simulink model "pure_pursuit_sl"  (R2019a)
settings: Solver=FixedStepDiscrete  StartTime=0.0  StopTime=inf  FixedStep=0.01  RelTol=1e-3
model workspace (MAT data in the model file):
  SL_ROS_VariableLengthArrays_MaxSizes : struct (value not decoded)
  MCOS : class17 (value not decoded)
  MCOS : class17 (value not decoded)
  MCOS : class17 (value not decoded)
  MCOS : class17 (value not decoded)
undefined symbols (not defined in the file): Action, Color, Colors, Colors_SL_Info, FrameLocked, Header, Id, Ns, Points, Points_SL_Info, Pose, Scale, Twist, Type, X, Y, Z
libraries: robotlib x22, robotcorelib x4, simulink x1
(part 2 of 2)

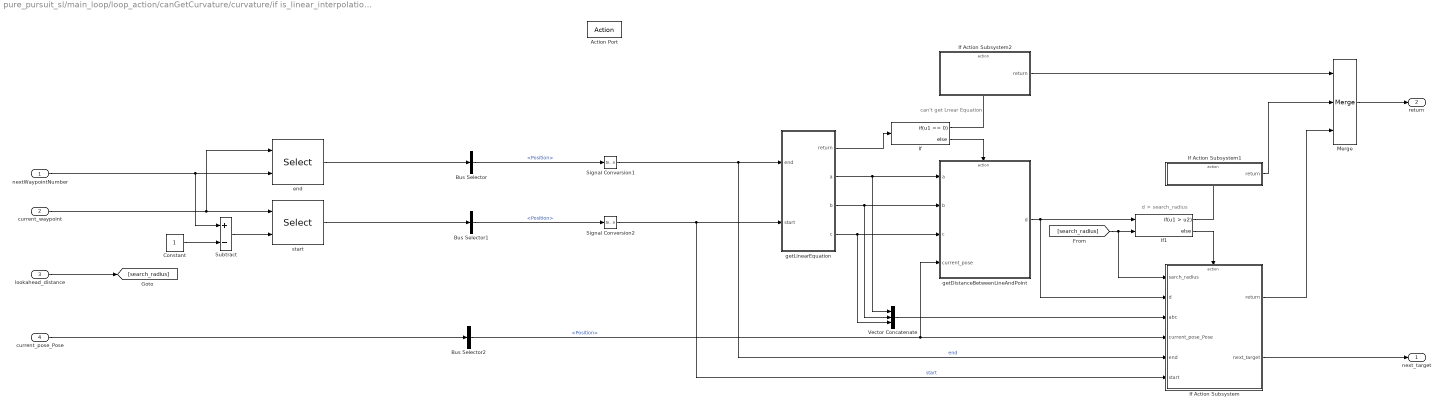
== system pure_pursuit_sl/main_loop/loop_action/canGetCurvature/curvature/if is_linear_interpolation_ is false or next waypoint is first or last/interpolateNextTarget/Subsystem ==
  note: d > search_radius
  note: can't get Lnear Equation
  nextWaypointNumber : Inport
  current_waypoint : Inport  Port=2
  lookahead_distance : Inport  Port=3
  current_pose_Pose : Inport  Port=4
  Action Port : ActionPort  ActionPortLabel=else
  Bus Selector : BusSelector  OutputSignals=Pose.Pose.Position
  Bus Selector1 : BusSelector  OutputSignals=Pose.Pose.Position
  Bus Selector2 : BusSelector  OutputSignals=Position
  Constant : Constant
  If : If  IfExpression=u1 == 0
  If Action Subsystem : Subsystem  TreatAsAtomicUnit=on
  If Action Subsystem1 : Subsystem  TreatAsAtomicUnit=on
  If Action Subsystem2 : Subsystem  TreatAsAtomicUnit=on
  If1 : If  NumInputs=2  IfExpression=u1 > u2
  Merge : Merge  Inputs=3
  Signal Conversion1 : SignalConversion  OverrideOpt=off
  Signal Conversion2 : SignalConversion  OverrideOpt=off
  Subtract : Sum  Inputs=+-
  Vector Concatenate : Concatenate  NumInputs=3
  end : Selector  InputPortWidth=101  IndexOptions=Index vector (port)  Indices=[1 3]  OutputSizes=1
  getDistanceBetweenLineAndPoint : Subsystem  TreatAsAtomicUnit=on
  getLinearEquation : Subsystem  TreatAsAtomicUnit=on
  start : Selector  InputPortWidth=101  IndexOptions=Index vector (port)  Indices=[1 3]  OutputSizes=1
  next_target : Outport
  return : Outport  Port=2
  wires:
  [search_radius] -> If Action Subsystem/1(sarch_radius), If1/2
  Bus Selector/1 -> Signal Conversion1/1  "<Position>"
  start/1 -> Bus Selector1/1
  If Action Subsystem/2(next_target) -> next_target/1
  Signal Conversion2/1 -> getLinearEquation/2(start), If Action Subsystem/6(start)  "start"
  getLinearEquation/3(b) -> Vector Concatenate/2, getDistanceBetweenLineAndPoint/2(b)
  If/2 -> getDistanceBetweenLineAndPoint/Action
  nextWaypointNumber/1 -> Subtract/1, end/2
  current_waypoint/1 -> end/1, start/1
  getDistanceBetweenLineAndPoint/1(d) -> If1/1, If Action Subsystem/2(d)
  Bus Selector2/1 -> getDistanceBetweenLineAndPoint/4(current_pose), If Action Subsystem/4(current_pose_Pose)  "<Position>"
  Merge/1 -> return/1
  If1/1 -> If Action Subsystem1/Action
  getLinearEquation/1(return) -> If/1
  getLinearEquation/4(c) -> Vector Concatenate/3, getDistanceBetweenLineAndPoint/3(c)
  Vector Concatenate/1 -> If Action Subsystem/3(abc)
  getLinearEquation/2(a) -> Vector Concatenate/1, getDistanceBetweenLineAndPoint/1(a)
  Signal Conversion1/1 -> getLinearEquation/1(end), If Action Subsystem/5(end)  "end"
  If1/2 -> If Action Subsystem/Action
  Subtract/1 -> start/2
  If Action Subsystem1/1(return) -> Merge/2
  Bus Selector1/1 -> Signal Conversion2/1  "<Position>"
  lookahead_distance/1 -> [search_radius]
  Constant/1 -> Subtract/2
  If/1 -> If Action Subsystem2/Action
  end/1 -> Bus Selector/1
  If Action Subsystem2/1(return) -> Merge/1
  If Action Subsystem/1(return) -> Merge/3
  current_pose_Pose/1 -> Bus Selector2/1

== system pure_pursuit_sl/main_loop/loop_action/canGetCurvature/curvature/if is_linear_interpolation_ is false or next waypoint is first or last/ next_waypoint_is_first_or_last/calcCurvature/calcRelativeCoordinate ==
  target : Inport
  current_pose_ : Inport  Port=2
  Bus Selector : BusSelector  OutputSignals=Orientation.W,Orientation.X,Orientation.Y,Orientation.Z
  Bus Selector1 : BusSelector  OutputSignals=Position.X,Position.Y,Position.Z
  Bus Selector3 : BusSelector  OutputSignals=X,Y,Z
  Constant : Constant
  Coordinate Transformation Conversion : robotcorelib/Coordinate Transformation Conversion  InputRepresentation=Quaternion  InputEulerSequence=XYZ  ShowTrVecInputPort=on  OutputRepresentation=Homogeneous Transformation  OutputEulerSequence=ZYX  ShowTrVecOutputPort=on  SimulateUsing=Interpreted execution
      settings: SourceProductBaseCode=RO
  Position Vector : Concatenate  NumInputs=3
  Product : Product  Inputs=/  Multiplication=Matrix(*)
  Product1 : Product  Multiplication=Matrix(*)
  "Quaternion Vector " : Concatenate  NumInputs=4
  point : Concatenate  NumInputs=4
  ros_pose : Outport
  wires:
  current_pose_/1 -> Bus Selector/1, Bus Selector1/1
  Position Vector/1 -> Coordinate Transformation Conversion/2
  Bus Selector1/3 -> Position Vector/3  "<Z>"
  "Quaternion Vector "/1 -> Coordinate Transformation Conversion/1
  Bus Selector1/2 -> Position Vector/2  "<Y>"
  Bus Selector1/1 -> Position Vector/1  "<X>"
  Coordinate Transformation Conversion/1 -> Product/1
  Product/1 -> Product1/1
  target/1 -> Bus Selector3/1
  Bus Selector3/2 -> point/2  "<Y>"
  Bus Selector3/3 -> point/3  "<Z>"
  Bus Selector3/1 -> point/1  "<X>"
  point/1 -> Product1/2
  Product1/1 -> ros_pose/1  "ros_pose"
  Bus Selector/1 -> "Quaternion Vector "/1  "<W>"
  Bus Selector/2 -> "Quaternion Vector "/2  "<X>"
  Bus Selector/3 -> "Quaternion Vector "/3  "<Y>"
  Bus Selector/4 -> "Quaternion Vector "/4  "<Z>"
  Constant/1 -> point/4

== system pure_pursuit_sl/main_loop/loop_action/canGetCurvature/curvature/if is_linear_interpolation_ is false or next waypoint is first or last/ next_waypoint_is_first_or_last/calcCurvature/getPlaneDistance ==
  target1 : Inport
  target2 : Inport  Port=2
  Add : Sum
  Bus Selector1 : BusSelector  OutputSignals=Position.X,Position.Y
  Bus Selector2 : BusSelector  OutputSignals=X,Y
  Math Function : Math  Operator=square  SaturateOnIntegerOverflow=on
  Math Function1 : Math  Operator=square  SaturateOnIntegerOverflow=on
  Sqrt : Sqrt  SaturateOnIntegerOverflow=on
  Subtract : Sum  Inputs=+-
  Subtract1 : Sum  Inputs=+-
  Distance : Outport
  wires:
  Subtract1/1 -> Math Function/1
  target2/1 -> Bus Selector1/1
  Bus Selector1/1 -> Subtract1/2  "<X>"
  target1/1 -> Bus Selector2/1
  Add/1 -> Sqrt/1
  Bus Selector2/1 -> Subtract1/1  "<X>"
  Bus Selector2/2 -> Subtract/1  "<Y>"
  Sqrt/1 -> Distance/1
  Math Function/1 -> Add/1
  Subtract/1 -> Math Function1/1
  Math Function1/1 -> Add/2
  Bus Selector1/2 -> Subtract/2  "<Y>"

== system pure_pursuit_sl/main_loop/loop_action/canGetCurvature/curvature/if is_linear_interpolation_ is false or next waypoint is first or last/ next_waypoint_is_first_or_last/calcCurvature/minus_KAPPA_MIN ==
  In1 : Inport
  Action Port : ActionPort  ActionPortLabel=else
  Unary Minus : UnaryMinus
  Out1 : Outport
  wires:
  In1/1 -> Unary Minus/1
  Unary Minus/1 -> Out1/1

== system pure_pursuit_sl/main_loop/loop_action/canGetCurvature/curvature/if is_linear_interpolation_ is false or next waypoint is first or last/ next_waypoint_is_first_or_last/calcCurvature/num_div_den ==
  denominator : Inport
  numerator : Inport  Port=2
  Action Port : ActionPort  ActionPortLabel=if(u1 ~= 0)
  Divide : Product  Inputs=*/
  kappa : Outport
  wires:
  denominator/1 -> Divide/2
  numerator/1 -> Divide/1
  Divide/1 -> kappa/1

== system pure_pursuit_sl/main_loop/loop_action/canGetCurvature/curvature/if is_linear_interpolation_ is false or next waypoint is first or last/ next_waypoint_is_first_or_last/calcCurvature/plus_KAPPA_MIN ==
  In1 : Inport
  Action Port : ActionPort  ActionPortLabel=elseif(u2 > 0)
  Out1 : Outport
  wires:
  In1/1 -> Out1/1

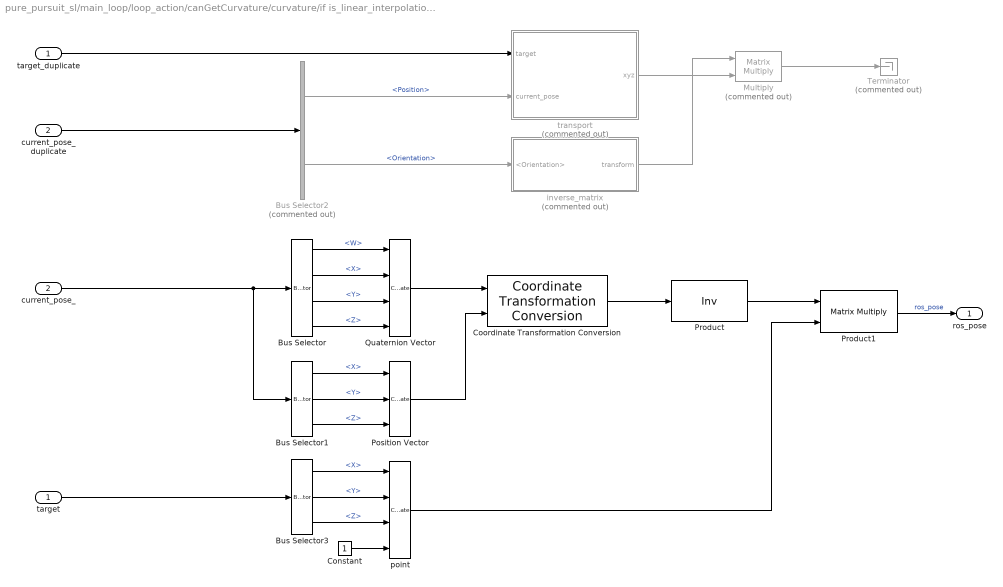
== system pure_pursuit_sl/main_loop/loop_action/canGetCurvature/curvature/if is_linear_interpolation_ is false or next waypoint is first or last/calcCurvature/calcCurvature/calcRelativeCoordinate ==
  target : Inport
  current_pose_ : Inport  Port=2
  Bus Selector : BusSelector  OutputSignals=Orientation.W,Orientation.X,Orientation.Y,Orientation.Z
  Bus Selector1 : BusSelector  OutputSignals=Position.X,Position.Y,Position.Z
  Bus Selector2 : BusSelector  Commented=on  OutputSignals=Position,Orientation
  Bus Selector3 : BusSelector  OutputSignals=X,Y,Z
  Constant : Constant
  Coordinate Transformation Conversion : robotcorelib/Coordinate Transformation Conversion  InputRepresentation=Quaternion  InputEulerSequence=XYZ  ShowTrVecInputPort=on  OutputRepresentation=Homogeneous Transformation  OutputEulerSequence=ZYX  ShowTrVecOutputPort=on  SimulateUsing=Interpreted execution
      settings: SourceProductBaseCode=RO
  Multiply : Product  Commented=on  Multiplication=Matrix(*)
  Position Vector : Concatenate  NumInputs=3
  Product : Product  Inputs=/  Multiplication=Matrix(*)
  Product1 : Product  Multiplication=Matrix(*)
  "Quaternion Vector " : Concatenate  NumInputs=4
  Terminator : Terminator  Commented=on
  current_pose_duplicate : InportShadow  Port=2
  inverse_matrix : Subsystem  Commented=on
  point : Concatenate  NumInputs=4
  target_duplicate : InportShadow
  transport : Subsystem  Commented=on
  ros_pose : Outport
  wires:
  Bus Selector2/2 -> inverse_matrix/1(<Orientation>)  "<Orientation>"
  transport/1(xyz) -> Multiply/2
  inverse_matrix/1(transform) -> Multiply/1
  target_duplicate/1 -> transport/1(target)
  Multiply/1 -> Terminator/1
  current_pose_/1 -> Bus Selector/1, Bus Selector1/1
  Bus Selector2/1 -> transport/2(current_pose)  "<Position>"
  Position Vector/1 -> Coordinate Transformation Conversion/2
  Bus Selector1/3 -> Position Vector/3  "<Z>"
  "Quaternion Vector "/1 -> Coordinate Transformation Conversion/1
  Bus Selector1/2 -> Position Vector/2  "<Y>"
  Bus Selector1/1 -> Position Vector/1  "<X>"
  Coordinate Transformation Conversion/1 -> Product/1
  current_pose_duplicate/1 -> Bus Selector2/1
  Product/1 -> Product1/1
  target/1 -> Bus Selector3/1
  Bus Selector3/2 -> point/2  "<Y>"
  Bus Selector3/3 -> point/3  "<Z>"
  Bus Selector3/1 -> point/1  "<X>"
  point/1 -> Product1/2
  Product1/1 -> ros_pose/1  "ros_pose"
  Bus Selector/1 -> "Quaternion Vector "/1  "<W>"
  Bus Selector/2 -> "Quaternion Vector "/2  "<X>"
  Bus Selector/3 -> "Quaternion Vector "/3  "<Y>"
  Bus Selector/4 -> "Quaternion Vector "/4  "<Z>"
  Constant/1 -> point/4

== system pure_pursuit_sl/main_loop/loop_action/canGetCurvature/curvature/if is_linear_interpolation_ is false or next waypoint is first or last/calcCurvature/calcCurvature/getPlaneDistance ==
  target1 : Inport
  target2 : Inport  Port=2
  Add : Sum
  Bus Selector1 : BusSelector  OutputSignals=Position.X,Position.Y
  Bus Selector2 : BusSelector  OutputSignals=X,Y
  Math Function : Math  Operator=square  SaturateOnIntegerOverflow=on
  Math Function1 : Math  Operator=square  SaturateOnIntegerOverflow=on
  Sqrt : Sqrt  SaturateOnIntegerOverflow=on
  Subtract : Sum  Inputs=+-
  Subtract1 : Sum  Inputs=+-
  Distance : Outport
  wires:
  Subtract1/1 -> Math Function/1
  target2/1 -> Bus Selector1/1
  Bus Selector1/1 -> Subtract1/2  "<X>"
  target1/1 -> Bus Selector2/1
  Add/1 -> Sqrt/1
  Bus Selector2/1 -> Subtract1/1  "<X>"
  Bus Selector2/2 -> Subtract/1  "<Y>"
  Sqrt/1 -> Distance/1
  Math Function/1 -> Add/1
  Subtract/1 -> Math Function1/1
  Math Function1/1 -> Add/2
  Bus Selector1/2 -> Subtract/2  "<Y>"

== system pure_pursuit_sl/main_loop/loop_action/canGetCurvature/curvature/if is_linear_interpolation_ is false or next waypoint is first or last/calcCurvature/calcCurvature/minus_KAPPA_MIN ==
  In1 : Inport
  Action Port : ActionPort  ActionPortLabel=else
  Unary Minus : UnaryMinus
  Out1 : Outport
  wires:
  In1/1 -> Unary Minus/1
  Unary Minus/1 -> Out1/1

== system pure_pursuit_sl/main_loop/loop_action/canGetCurvature/curvature/if is_linear_interpolation_ is false or next waypoint is first or last/calcCurvature/calcCurvature/num_div_den ==
  denominator : Inport
  numerator : Inport  Port=2
  Action Port : ActionPort  ActionPortLabel=if(u1 ~= 0)
  Divide : Product  Inputs=*/
  kappa : Outport
  wires:
  denominator/1 -> Divide/2
  numerator/1 -> Divide/1
  Divide/1 -> kappa/1

== system pure_pursuit_sl/main_loop/loop_action/canGetCurvature/curvature/if is_linear_interpolation_ is false or next waypoint is first or last/calcCurvature/calcCurvature/plus_KAPPA_MIN ==
  In1 : Inport
  Action Port : ActionPort  ActionPortLabel=elseif(u2 > 0)
  Out1 : Outport
  wires:
  In1/1 -> Out1/1

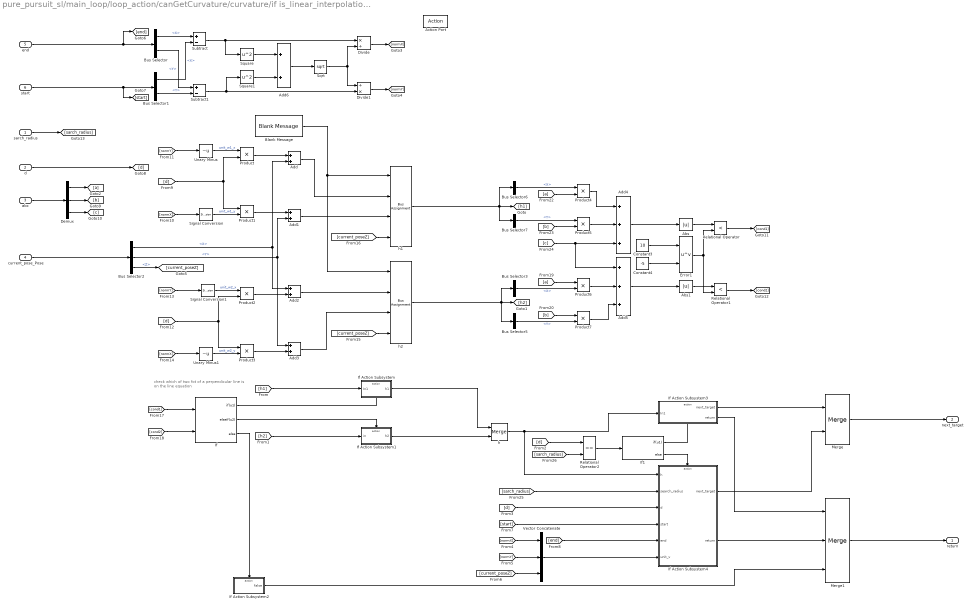
== system pure_pursuit_sl/main_loop/loop_action/canGetCurvature/curvature/if is_linear_interpolation_ is false or next waypoint is first or last/interpolateNextTarget/Subsystem/If Action Subsystem ==
  note: check which of two fot of a perpendicular line
      | is on the line equation
  sarch_radius : Inport
  d : Inport  Port=2
  abc : Inport  Port=3
  current_pose_Pose : Inport  Port=4
  end : Inport  Port=5
  start : Inport  Port=6
  Action Port : ActionPort  ActionPortLabel=else
  Abs : Abs
  Abs1 : Abs
  Add{,1..3,6} (5 alike) : Sum
  Add4 : Sum  Inputs=+++
  Add5 : Sum  Inputs=+++
  Blank Message : robotlib/Blank Message  messageClass=Message  entityType=geometry_msgs/Point  messageType=geometry_msgs/Point  SampleTime=inf
      settings: SourceProductBaseCode=RO
  Bus Selector : BusSelector  OutputSignals=X,Y
  Bus Selector1 : BusSelector  OutputSignals=X,Y
  Bus Selector2 : BusSelector  OutputSignals=X,Y,Z
  Bus Selector3 : BusSelector  OutputSignals=X
  Bus Selector5 : BusSelector  OutputSignals=Y
  Bus Selector6 : BusSelector  OutputSignals=X
  Bus Selector7 : BusSelector  OutputSignals=Y
  Constant3 : Constant  Value=10  OutDataTypeStr=double
  Constant4 : Constant  Value=-5  OutDataTypeStr=double
  Demux : Demux  Outputs=3
  Divide : Product  Inputs=*/
  Divide1 : Product  Inputs=/*
  Error1 : Math  Operator=pow  SaturateOnIntegerOverflow=on
  If : If  NumInputs=2  IfExpression=u1  ElseIfExpressions=u2
  If Action Subsystem : Subsystem  TreatAsAtomicUnit=on
  If Action Subsystem1 : Subsystem  TreatAsAtomicUnit=on
  If Action Subsystem2 : Subsystem  TreatAsAtomicUnit=on
  If Action Subsystem3 : Subsystem  TreatAsAtomicUnit=on
  If Action Subsystem4 : Subsystem  Description=|  TreatAsAtomicUnit=on
      | if there are two intersection
      | get intersection in front of vehicle
      settings: AttributesFormatString=%<Description>
  If1 : If  IfExpression=u1
  Merge : Merge
  Merge1 : Merge  Inputs=3
  Product{,1..7} (8 alike) : Product
  Relational Operator : RelationalOperator  Operator=<  OutDataTypeStr=boolean  RndMeth=Simplest
  Relational Operator1 : RelationalOperator  Operator=<  OutDataTypeStr=boolean  RndMeth=Simplest
  Relational Operator2 : RelationalOperator  Operator===  OutDataTypeStr=boolean  RndMeth=Simplest
  Signal Conversion : SignalConversion  OverrideOpt=off
  Signal Conversion1 : SignalConversion  OverrideOpt=off
  Sqrt : Sqrt  SaturateOnIntegerOverflow=on
  Square : Math  Operator=square  SaturateOnIntegerOverflow=on
  Square1 : Math  Operator=square  SaturateOnIntegerOverflow=on
  Subtract : Sum  Inputs=+-
  Subtract1 : Sum  Inputs=+-
  Unary Minus : UnaryMinus
  Unary Minus1 : UnaryMinus
  Vector Concatenate : Concatenate  NumInputs=3
  h : Merge
  h1 : BusAssignment  AssignedSignals=X,Y,Z
  h2 : BusAssignment  AssignedSignals=X,Y,Z
  return : Outport
  next_target : Outport  Port=2
  wires:
  Bus Selector/2 -> Subtract1/1  "<Y>"
  end/1 -> [end], Bus Selector/1
  start/1 -> [start], Bus Selector1/1
  Bus Selector/1 -> Subtract/1  "<X>"
  Bus Selector1/1 -> Subtract/2  "<X>"
  Bus Selector1/2 -> Subtract1/2  "<Y>"
  [normX] -> Signal Conversion/1
  [normY] -> Unary Minus/1
  Unary Minus/1 -> Product/1  "unit_w1_x"
  current_pose_Pose/1 -> Bus Selector2/1
  Bus Selector2/1 -> Add2/1, Add/2  "<X>"
  Blank Message/1 -> h1/1, h2/1
  Bus Selector2/3 -> [current_poseZ]  "<Z>"
  Product/1 -> Add/1
  [d] -> Product1/1, Product/2
  Product1/1 -> Add1/1
  Bus Selector2/2 -> Add3/1, Add1/2  "<Y>"
  Product2/1 -> Add2/2
  Product3/1 -> Add3/2
  Add/1 -> h1/2
  Add1/1 -> h1/3
  Add2/1 -> h2/2
  Add3/1 -> h2/3
  Bus Selector6/1 -> Product4/1  "<X>"
  [a] -> Product6/1
  Bus Selector7/1 -> Product5/1  "<Y>"
  [b] -> Product7/1
  Product4/1 -> Add4/1
  Product5/1 -> Add4/2
  [c] -> Add5/1, Add4/3
  Bus Selector3/1 -> Product6/2  "<X>"
  Bus Selector5/1 -> Product7/2  "<Y>"
  Product6/1 -> Add5/2
  Product7/1 -> Add5/3
  Constant4/1 -> Error1/2
  Constant3/1 -> Error1/1
  Add4/1 -> Abs/1
  Add5/1 -> Abs1/1
  If/1 -> If Action Subsystem/Action
  If/2 -> If Action Subsystem1/Action
  [h1] -> If Action Subsystem/1(In1)
  [h2] -> If Action Subsystem1/1(in)
  If/3 -> If Action Subsystem2/Action
  If Action Subsystem/1(h1) -> h/1
  If Action Subsystem1/1("h2 ") -> h/2
  sarch_radius/1 -> [sarch_radius]
  [d] -> Relational Operator2/1
  If1/1 -> If Action Subsystem3/Action
  h/1 -> If Action Subsystem3/1(In1), If Action Subsystem4/1(h)
  If1/2 -> If Action Subsystem4/Action
  [d] -> If Action Subsystem4/3(d)
  [normY] -> Vector Concatenate/2
  [normX] -> Vector Concatenate/1
  [current_poseZ] -> Vector Concatenate/3
  Vector Concatenate/1 -> If Action Subsystem4/6(unit_v)
  [start] -> If Action Subsystem4/4(start)
  [end] -> If Action Subsystem4/5("end ")
  If Action Subsystem3/1(next_target) -> Merge/1
  If Action Subsystem4/1(next_target) -> Merge/2
  If Action Subsystem4/2(return) -> Merge1/2
  If Action Subsystem3/2(return) -> Merge1/1
  If Action Subsystem2/1(false) -> Merge1/3
  Merge/1 -> next_target/1
  Merge1/1 -> return/1
  d/1 -> [d]
  Subtract1/1 -> Square1/1, Divide1/2
  Square/1 -> Add6/1
  Subtract/1 -> Square/1, Divide/1
  Square1/1 -> Add6/2
  Add6/1 -> Sqrt/1
  Sqrt/1 -> Divide/2, Divide1/1
  Divide/1 -> [normX]
  Divide1/1 -> [normY]
  Signal Conversion/1 -> Product1/2  "unit_w1_y"
  [d] -> Product3/1, Product2/2
  Unary Minus1/1 -> Product3/2  "unit_w2_y"
  Signal Conversion1/1 -> Product2/1  "unit_w2_x"
  [normY] -> Signal Conversion1/1
  [normX] -> Unary Minus1/1
  [current_poseZ] -> h2/4
  [current_poseZ] -> h1/4
  h1/1 -> Bus Selector6/1, Bus Selector7/1, [h1]
  abc/1 -> Demux/1
  Demux/1 -> [a]
  Demux/2 -> [b]
  Demux/3 -> [c]
  [a] -> Product4/2
  [b] -> Product5/2
  h2/1 -> Bus Selector5/1, [h2], Bus Selector3/1
  Abs/1 -> Relational Operator/1
  Error1/1 -> Relational Operator1/2, Relational Operator/2
  Abs1/1 -> Relational Operator1/1
  Relational Operator/1 -> [cond1]
  Relational Operator1/1 -> [cond2]
  [cond1] -> If/1
  [cond2] -> If/2
  [sarch_radius] -> If Action Subsystem4/2(search_radius)
  [sarch_radius] -> Relational Operator2/2
  Relational Operator2/1 -> If1/1

== system pure_pursuit_sl/main_loop/loop_action/canGetCurvature/curvature/if is_linear_interpolation_ is false or next waypoint is first or last/interpolateNextTarget/Subsystem/If Action Subsystem1 ==
  Action Port : ActionPort  ActionPortLabel=if(u1 > u2)
  Constant1 : Constant  Value=false  OutDataTypeStr=boolean
  return : Outport  InitialOutput=false
  wires:
  Constant1/1 -> return/1

== system pure_pursuit_sl/main_loop/loop_action/canGetCurvature/curvature/if is_linear_interpolation_ is false or next waypoint is first or last/interpolateNextTarget/Subsystem/If Action Subsystem2 ==
  Action Port : ActionPort  ActionPortLabel=if(u1 == 0)
  Constant1 : Constant  Value=false  OutDataTypeStr=boolean
  return : Outport  InitialOutput=false
  wires:
  Constant1/1 -> return/1

== system pure_pursuit_sl/main_loop/loop_action/canGetCurvature/curvature/if is_linear_interpolation_ is false or next waypoint is first or last/interpolateNextTarget/Subsystem/getDistanceBetweenLineAndPoint ==
  a : Inport
  b : Inport  Port=2
  c : Inport  Port=3
  current_pose : Inport  Port=4
  Action Port : ActionPort  ActionPortLabel=else
  Abs : Abs
  Add : Sum  Inputs=+++
  Add1 : Sum
  Bus Selector1 : BusSelector  OutputSignals=X,Y
  Divide : Product  Inputs=*/
  Product : Product
  Product1 : Product
  Sqrt : Sqrt  SaturateOnIntegerOverflow=on
  Square : Math  Operator=square  SaturateOnIntegerOverflow=on
  Square1 : Math  Operator=square  SaturateOnIntegerOverflow=on
  d : Outport
  wires:
  a/1 -> Product/2, Square/1
  current_pose/1 -> Bus Selector1/1
  Bus Selector1/1 -> Product/1  "<X>"
  b/1 -> Product1/2, Square1/1
  Bus Selector1/2 -> Product1/1  "<Y>"
  Product/1 -> Add/2
  Product1/1 -> Add/3
  Add1/1 -> Sqrt/1
  Square/1 -> Add1/1
  Square1/1 -> Add1/2
  Add/1 -> Abs/1
  Sqrt/1 -> Divide/2
  Divide/1 -> d/1
  Abs/1 -> Divide/1
  c/1 -> Add/1

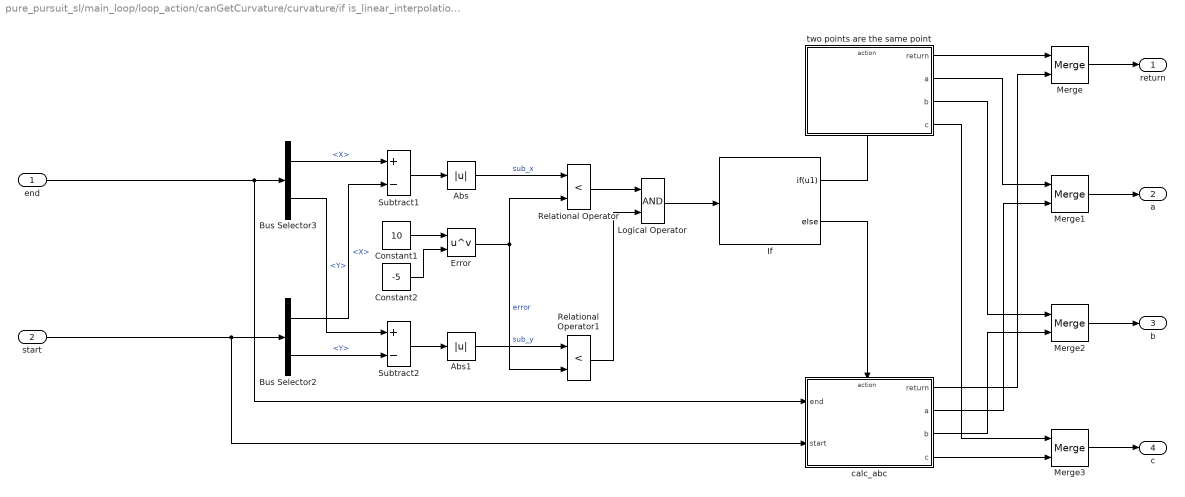
== system pure_pursuit_sl/main_loop/loop_action/canGetCurvature/curvature/if is_linear_interpolation_ is false or next waypoint is first or last/interpolateNextTarget/Subsystem/getLinearEquation ==
  end : Inport
  start : Inport  Port=2
  Abs : Abs
  Abs1 : Abs
  Bus Selector2 : BusSelector  OutputSignals=X,Y
  Bus Selector3 : BusSelector  OutputSignals=X,Y
  Constant1 : Constant  Value=10  OutDataTypeStr=double
  Constant2 : Constant  Value=-5  OutDataTypeStr=double
  Error : Math  Operator=pow  SaturateOnIntegerOverflow=on
  If : If  IfExpression=u1
  Logical Operator : Logic  AllPortsSameDT=off  OutDataTypeStr=boolean
  Merge{,1..3} (4 alike) : Merge
  Relational Operator : RelationalOperator  Operator=<  OutDataTypeStr=boolean  RndMeth=Simplest
  Relational Operator1 : RelationalOperator  Operator=<  OutDataTypeStr=boolean  RndMeth=Simplest
  Subtract1 : Sum  Inputs=+-
  Subtract2 : Sum  Inputs=+-
  calc_abc : Subsystem  TreatAsAtomicUnit=on
  two points are the same point : Subsystem  TreatAsAtomicUnit=on
  return : Outport
  a : Outport  Port=2
  b : Outport  Port=3
  c : Outport  Port=4
  wires:
  Error/1 -> Relational Operator1/2, Relational Operator/2  "error"
  two points are the same point/1(return) -> Merge/1
  Bus Selector3/2 -> Subtract2/1  "<Y>"
  If/2 -> calc_abc/Action
  Merge/1 -> return/1
  Abs1/1 -> Relational Operator1/1  "sub_y"
  Bus Selector2/1 -> Subtract1/2  "<X>"
  Abs/1 -> Relational Operator/1  "sub_x"
  Subtract1/1 -> Abs/1
  calc_abc/1(return) -> Merge/2
  If/1 -> two points are the same point/Action
  start/1 -> Bus Selector2/1, calc_abc/2(start)
  Bus Selector3/1 -> Subtract1/1  "<X>"
  Subtract2/1 -> Abs1/1
  Bus Selector2/2 -> Subtract2/2  "<Y>"
  end/1 -> Bus Selector3/1, calc_abc/1(end)
  Constant2/1 -> Error/2
  Constant1/1 -> Error/1
  Relational Operator/1 -> Logical Operator/1
  Relational Operator1/1 -> Logical Operator/2
  Logical Operator/1 -> If/1
  Merge3/1 -> c/1
  calc_abc/4(c) -> Merge3/2
  two points are the same point/4(c) -> Merge3/1
  two points are the same point/2(a) -> Merge1/1
  calc_abc/2(a) -> Merge1/2
  Merge1/1 -> a/1
  Merge2/1 -> b/1
  two points are the same point/3(b) -> Merge2/1
  calc_abc/3(b) -> Merge2/2

== system pure_pursuit_sl/main_loop/loop_action/canGetCurvature/curvature/if is_linear_interpolation_ is false or next waypoint is first or last/calcCurvature/calcCurvature/calcRelativeCoordinate/inverse_matrix ==
  <Orientation> : Inport
  Bus Creator : BusCreator  Inputs=4
  Bus Selector1 : BusSelector  OutputSignals=W,X,Y,Z
  Bus to Vector : BusToVector
  Coordinate Transformation Conversion : robotcorelib/Coordinate Transformation Conversion  InputRepresentation=Quaternion  InputEulerSequence=ZYX  ShowTrVecInputPort=on  OutputRepresentation=Rotation Matrix  OutputEulerSequence=ZYX  ShowTrVecOutputPort=on  SimulateUsing=Interpreted execution
      settings: SourceProductBaseCode=RO
  inverse : MATLAB Function  TreatAsAtomicUnit=on
  transform : Outport
  wires:
  Coordinate Transformation Conversion/1 -> inverse/1(u)
  inverse/1(y) -> transform/1
  Bus Selector1/3 -> Bus Creator/3  "<Y>"
  Bus Creator/1 -> Bus to Vector/1
  <Orientation>/1 -> Bus Selector1/1
  Bus to Vector/1 -> Coordinate Transformation Conversion/1
  Bus Selector1/1 -> Bus Creator/1  "<W>"
  Bus Selector1/4 -> Bus Creator/4  "<Z>"
  Bus Selector1/2 -> Bus Creator/2  "<X>"

== system pure_pursuit_sl/main_loop/loop_action/canGetCurvature/curvature/if is_linear_interpolation_ is false or next waypoint is first or last/calcCurvature/calcCurvature/calcRelativeCoordinate/transport ==
  target : Inport
  current_pose : Inport  Port=2
  Bus Creator1 : BusCreator  Inputs=3
  Bus Selector3 : BusSelector  OutputSignals=X,Y,Z
  Bus Selector4 : BusSelector  OutputSignals=X,Y,Z
  Bus to Vector1 : BusToVector
  Subtract : Sum  Inputs=+-
  Subtract1 : Sum  Inputs=+-
  Subtract2 : Sum  Inputs=+-
  xyz : Outport
  wires:
  Bus Selector3/2 -> Subtract2/2  "<Y>"
  Bus Selector4/3 -> Subtract1/1  "<Z>"
  Bus Selector4/1 -> Subtract/1  "<X>"
  Bus Selector3/3 -> Subtract1/2  "<Z>"
  target/1 -> Bus Selector4/1
  Subtract1/1 -> Bus Creator1/3
  Bus Selector4/2 -> Subtract2/1  "<Y>"
  Bus Creator1/1 -> Bus to Vector1/1
  Bus to Vector1/1 -> xyz/1
  Subtract/1 -> Bus Creator1/1
  current_pose/1 -> Bus Selector3/1
  Subtract2/1 -> Bus Creator1/2
  Bus Selector3/1 -> Subtract/2  "<X>"

== system pure_pursuit_sl/main_loop/loop_action/canGetCurvature/curvature/if is_linear_interpolation_ is false or next waypoint is first or last/interpolateNextTarget/Subsystem/If Action Subsystem/If Action Subsystem ==
  In1 : Inport
  Action Port : ActionPort  ActionPortLabel=if(u1)
  h1 : Outport
  wires:
  In1/1 -> h1/1

== system pure_pursuit_sl/main_loop/loop_action/canGetCurvature/curvature/if is_linear_interpolation_ is false or next waypoint is first or last/interpolateNextTarget/Subsystem/If Action Subsystem/If Action Subsystem1 ==
  in : Inport
  Action Port : ActionPort  ActionPortLabel=elseif(u2)
  "h2 " : Outport
  wires:
  in/1 -> "h2 "/1

== system pure_pursuit_sl/main_loop/loop_action/canGetCurvature/curvature/if is_linear_interpolation_ is false or next waypoint is first or last/interpolateNextTarget/Subsystem/If Action Subsystem/If Action Subsystem2 ==
  Action Port : ActionPort  ActionPortLabel=else
  Constant1 : Constant  Value=false  OutDataTypeStr=boolean
  false : Outport  InitialOutput=false
  wires:
  Constant1/1 -> false/1

== system pure_pursuit_sl/main_loop/loop_action/canGetCurvature/curvature/if is_linear_interpolation_ is false or next waypoint is first or last/interpolateNextTarget/Subsystem/If Action Subsystem/If Action Subsystem3 ==
  In1 : Inport
  Action Port : ActionPort  ActionPortLabel=if(u1)
  Constant1 : Constant  Value=true  OutDataTypeStr=boolean
  next_target : Outport
  return : Outport  Port=2  InitialOutput=true
  wires:
  In1/1 -> next_target/1
  Constant1/1 -> return/1

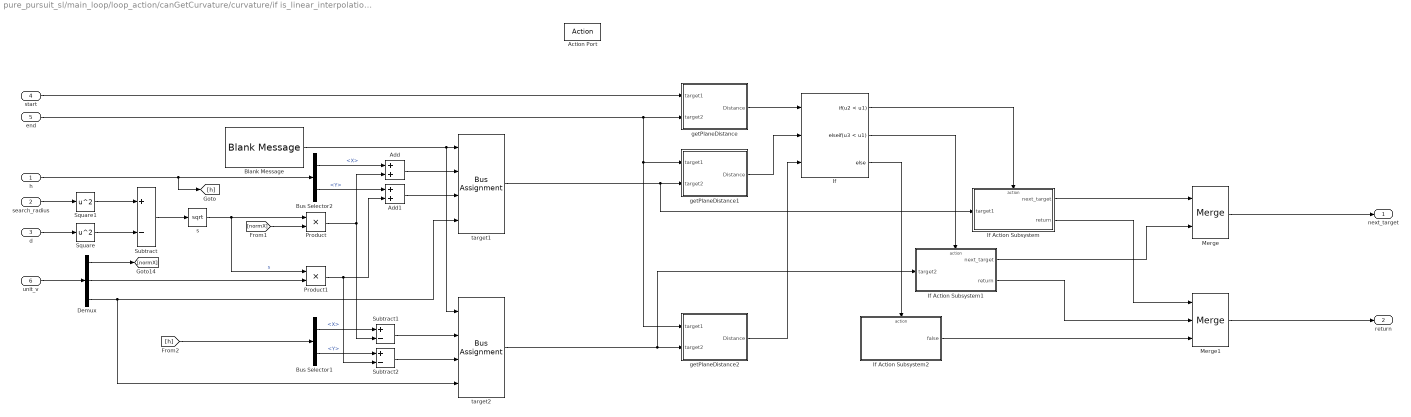
== system pure_pursuit_sl/main_loop/loop_action/canGetCurvature/curvature/if is_linear_interpolation_ is false or next waypoint is first or last/interpolateNextTarget/Subsystem/If Action Subsystem/If Action Subsystem4 ==
  h : Inport
  search_radius : Inport  Port=2
  d : Inport  Port=3
  start : Inport  Port=4
  "end " : Inport  Port=5
  unit_v : Inport  Port=6
  Action Port : ActionPort  ActionPortLabel=else
  Add : Sum
  Add1 : Sum
  Blank Message : robotlib/Blank Message  messageClass=Message  entityType=geometry_msgs/Point  messageType=geometry_msgs/Point  SampleTime=inf
      settings: SourceProductBaseCode=RO
  Bus Selector1 : BusSelector  OutputSignals=X,Y
  Bus Selector2 : BusSelector  OutputSignals=X,Y
  Demux : Demux  Outputs=3
  If : If  NumInputs=3  IfExpression=u2 < u1  ElseIfExpressions=u3 < u1
  If Action Subsystem : Subsystem  TreatAsAtomicUnit=on
  If Action Subsystem1 : Subsystem  TreatAsAtomicUnit=on
  If Action Subsystem2 : Subsystem  TreatAsAtomicUnit=on
  Merge : Merge
  Merge1 : Merge  Inputs=3
  Product : Product
  Product1 : Product
  Square : Math  Operator=square  SaturateOnIntegerOverflow=on
  Square1 : Math  Operator=square  SaturateOnIntegerOverflow=on
  Subtract : Sum  Inputs=+-
  Subtract1 : Sum  Inputs=+-
  Subtract2 : Sum  Inputs=+-
  getPlaneDistance : Subsystem  TreatAsAtomicUnit=on
  getPlaneDistance1 : Subsystem  TreatAsAtomicUnit=on
  getPlaneDistance2 : Subsystem  TreatAsAtomicUnit=on
  s : Sqrt  SaturateOnIntegerOverflow=on
  target1 : BusAssignment  AssignedSignals=X,Y,Z
  target2 : BusAssignment  AssignedSignals=X,Y,Z
  next_target : Outport
  return : Outport  Port=2
  wires:
  Subtract/1 -> s/1
  d/1 -> Square/1
  search_radius/1 -> Square1/1
  Square1/1 -> Subtract/1
  Square/1 -> Subtract/2
  s/1 -> Product/1, Product1/1  "s"
  Blank Message/1 -> target2/1, target1/1
  unit_v/1 -> Demux/1
  Demux/1 -> [normX]
  Demux/2 -> Product1/2
  Demux/3 -> target1/4, target2/4
  Bus Selector2/1 -> Add/1  "<X>"
  Product/1 -> Add/2, Subtract1/2
  Add/1 -> target1/2
  Add1/1 -> target1/3
  Product1/1 -> Subtract2/2, Add1/2
  Subtract1/1 -> target2/2
  Subtract2/1 -> target2/3
  target1/1 -> getPlaneDistance1/2(target2), If Action Subsystem/1(target1)
  target2/1 -> getPlaneDistance2/2(target2), If Action Subsystem1/1(target2)
  start/1 -> getPlaneDistance/1(target1)
  "end "/1 -> getPlaneDistance/2(target2), getPlaneDistance1/1(target1), getPlaneDistance2/1(target1)
  getPlaneDistance/1(Distance) -> If/1
  getPlaneDistance1/1(Distance) -> If/2
  getPlaneDistance2/1(Distance) -> If/3
  If/1 -> If Action Subsystem/Action
  If/2 -> If Action Subsystem1/Action
  If/3 -> If Action Subsystem2/Action
  If Action Subsystem/1(next_target) -> Merge/1
  If Action Subsystem1/1(next_target) -> Merge/2
  If Action Subsystem/2(return) -> Merge1/1
  Merge1/1 -> return/1
  If Action Subsystem1/2(return) -> Merge1/2
  If Action Subsystem2/1(false) -> Merge1/3
  Merge/1 -> next_target/1
  h/1 -> Bus Selector2/1, [h]
  [h] -> Bus Selector1/1
  [normX] -> Product/2
  Bus Selector2/2 -> Add1/1  "<Y>"
  Bus Selector1/1 -> Subtract1/1  "<X>"
  Bus Selector1/2 -> Subtract2/1  "<Y>"

== system pure_pursuit_sl/main_loop/loop_action/canGetCurvature/curvature/if is_linear_interpolation_ is false or next waypoint is first or last/interpolateNextTarget/Subsystem/getLinearEquation/calc_abc ==
  end : Inport
  start : Inport  Port=2
  Action Port : ActionPort  ActionPortLabel=else
  Add : Sum
  Bus Selector : BusSelector  OutputSignals=Y,X
  Bus Selector1 : BusSelector  OutputSignals=Y,X
  Constant2 : Constant  Value=true  OutDataTypeStr=boolean
  Gain : Gain  Gain=-1
  Gain1 : Gain  Gain=-1
  Product2 : Product
  Product3 : Product
  Subtract : Sum  Inputs=+-
  Subtract1 : Sum  Inputs=+-
  return : Outport
  a : Outport  Port=2
  b : Outport  Port=3
  c : Outport  Port=4
  wires:
  end/1 -> Bus Selector/1
  start/1 -> Bus Selector1/1
  Bus Selector/2 -> Subtract1/1  "<X>"
  Bus Selector/1 -> Subtract/1  "<Y>"
  Bus Selector1/2 -> Subtract1/2, Product2/2  "<X>"
  Bus Selector1/1 -> Subtract/2, Product3/2  "<Y>"
  Subtract1/1 -> Gain/1, Product3/1
  Gain/1 -> b/1
  Subtract/1 -> Gain1/1, a/1
  Product3/1 -> Add/1
  Product2/1 -> Add/2
  Add/1 -> c/1
  Constant2/1 -> return/1
  Gain1/1 -> Product2/1

== system pure_pursuit_sl/main_loop/loop_action/canGetCurvature/curvature/if is_linear_interpolation_ is false or next waypoint is first or last/interpolateNextTarget/Subsystem/getLinearEquation/two points are the same point ==
  Action Port : ActionPort  ActionPortLabel=if(u1)
  Constant : Constant  Value=0
  Constant1 : Constant  Value=false  OutDataTypeStr=boolean
  return : Outport  InitialOutput=false
  a : Outport  Port=2
  b : Outport  Port=3
  c : Outport  Port=4
  wires:
  Constant1/1 -> return/1
  Constant/1 -> b/1, c/1, a/1

== system pure_pursuit_sl/main_loop/loop_action/canGetCurvature/curvature/if is_linear_interpolation_ is false or next waypoint is first or last/interpolateNextTarget/Subsystem/If Action Subsystem/If Action Subsystem4/If Action Subsystem ==
  target1 : Inport
  Action Port : ActionPort  ActionPortLabel=if(u2 < u1)
  Constant1 : Constant  Value=true  OutDataTypeStr=boolean
  next_target : Outport
  return : Outport  Port=2  InitialOutput=true
  wires:
  target1/1 -> next_target/1
  Constant1/1 -> return/1

== system pure_pursuit_sl/main_loop/loop_action/canGetCurvature/curvature/if is_linear_interpolation_ is false or next waypoint is first or last/interpolateNextTarget/Subsystem/If Action Subsystem/If Action Subsystem4/If Action Subsystem1 ==
  target2 : Inport
  Action Port : ActionPort  ActionPortLabel=elseif(u3 < u1)
  Constant1 : Constant  Value=true  OutDataTypeStr=boolean
  next_target : Outport
  return : Outport  Port=2  InitialOutput=true
  wires:
  target2/1 -> next_target/1
  Constant1/1 -> return/1

== system pure_pursuit_sl/main_loop/loop_action/canGetCurvature/curvature/if is_linear_interpolation_ is false or next waypoint is first or last/interpolateNextTarget/Subsystem/If Action Subsystem/If Action Subsystem4/If Action Subsystem2 ==
  Action Port : ActionPort  ActionPortLabel=else
  Constant1 : Constant  Value=false  OutDataTypeStr=boolean
  false : Outport  InitialOutput=false
  wires:
  Constant1/1 -> false/1

== system pure_pursuit_sl/main_loop/loop_action/canGetCurvature/curvature/if is_linear_interpolation_ is false or next waypoint is first or last/interpolateNextTarget/Subsystem/If Action Subsystem/If Action Subsystem4/getPlaneDistance ==
  target1 : Inport
  target2 : Inport  Port=2
  Add : Sum
  Bus Selector1 : BusSelector  OutputSignals=X,Y
  Bus Selector2 : BusSelector  OutputSignals=X,Y
  Math Function : Math  Operator=square  SaturateOnIntegerOverflow=on
  Math Function1 : Math  Operator=square  SaturateOnIntegerOverflow=on
  Sqrt : Sqrt  SaturateOnIntegerOverflow=on
  Subtract : Sum  Inputs=+-
  Subtract1 : Sum  Inputs=+-
  Distance : Outport
  wires:
  Subtract1/1 -> Math Function/1
  target2/1 -> Bus Selector1/1
  Bus Selector1/1 -> Subtract1/2  "<X>"
  target1/1 -> Bus Selector2/1
  Add/1 -> Sqrt/1
  Bus Selector2/1 -> Subtract1/1  "<X>"
  Bus Selector2/2 -> Subtract/1  "<Y>"
  Sqrt/1 -> Distance/1
  Math Function/1 -> Add/1
  Subtract/1 -> Math Function1/1
  Math Function1/1 -> Add/2
  Bus Selector1/2 -> Subtract/2  "<Y>"

== system pure_pursuit_sl/main_loop/loop_action/canGetCurvature/curvature/if is_linear_interpolation_ is false or next waypoint is first or last/interpolateNextTarget/Subsystem/If Action Subsystem/If Action Subsystem4/getPlaneDistance1 ==
  target1 : Inport
  target2 : Inport  Port=2
  Add : Sum
  Bus Selector1 : BusSelector  OutputSignals=X,Y
  Bus Selector2 : BusSelector  OutputSignals=X,Y
  Math Function : Math  Operator=square  SaturateOnIntegerOverflow=on
  Math Function1 : Math  Operator=square  SaturateOnIntegerOverflow=on
  Sqrt : Sqrt  SaturateOnIntegerOverflow=on
  Subtract : Sum  Inputs=+-
  Subtract1 : Sum  Inputs=+-
  Distance : Outport
  wires:
  Bus Selector1/2 -> Subtract/2  "<Y>"
  Math Function1/1 -> Add/2
  Subtract/1 -> Math Function1/1
  Math Function/1 -> Add/1
  Sqrt/1 -> Distance/1
  Bus Selector2/2 -> Subtract/1  "<Y>"
  Bus Selector2/1 -> Subtract1/1  "<X>"
  Add/1 -> Sqrt/1
  target1/1 -> Bus Selector2/1
  Bus Selector1/1 -> Subtract1/2  "<X>"
  target2/1 -> Bus Selector1/1
  Subtract1/1 -> Math Function/1

== system pure_pursuit_sl/main_loop/loop_action/canGetCurvature/curvature/if is_linear_interpolation_ is false or next waypoint is first or last/interpolateNextTarget/Subsystem/If Action Subsystem/If Action Subsystem4/getPlaneDistance2 ==
  target1 : Inport
  target2 : Inport  Port=2
  Add : Sum
  Bus Selector1 : BusSelector  OutputSignals=X,Y
  Bus Selector2 : BusSelector  OutputSignals=X,Y
  Math Function : Math  Operator=square  SaturateOnIntegerOverflow=on
  Math Function1 : Math  Operator=square  SaturateOnIntegerOverflow=on
  Sqrt : Sqrt  SaturateOnIntegerOverflow=on
  Subtract : Sum  Inputs=+-
  Subtract1 : Sum  Inputs=+-
  Distance : Outport
  wires:
  Bus Selector1/2 -> Subtract/2  "<Y>"
  Math Function1/1 -> Add/2
  Subtract/1 -> Math Function1/1
  Math Function/1 -> Add/1
  Sqrt/1 -> Distance/1
  Bus Selector2/2 -> Subtract/1  "<Y>"
  Bus Selector2/1 -> Subtract1/1  "<X>"
  Add/1 -> Sqrt/1
  target1/1 -> Bus Selector2/1
  Bus Selector1/1 -> Subtract1/2  "<X>"
  target2/1 -> Bus Selector1/1
  Subtract1/1 -> Math Function/1

== matlab function pure_pursuit_sl/main_loop/loop_action/VisualizationWithRviz/generateTrajectoryCircle/MATLAB Function ==
  data: blank_msg input Bus: SL_Bus_pure_pursuit_sl_geometry_msgs_Point; radius input; traj_circle_array output Bus: SL_Bus_pure_pursuit_sl_geometry_msgs_Point size=80; current_pose input
function traj_circle_array = fcn(blank_msg, radius, current_pose)
% 

% traj_circle_array = zeros(80, 1);
% traj_circle_array = struct([]);   NG
traj_circle_array = repmat(blank_msg, 80, 1);
range = pi() / 8;
increment = 0.01;
idx = 1;

for rad = 0:increment:range
    % calc a point of circumference
    p = blank_msg;
    p.X = radius * cos(rad);
    p.Y = radius * sin(rad);
    
    % transform to (radius,0)
    relative_p = blank_msg;
    relative_p.X = p.X - radius;
    relative_p.Y = p.Y;

    % rotate -90°
    rotate_p = autoware.LibWaypointFollower.rotatePoint(relative_p, -90);

    % transform to vehicle plane
    tf_p = autoware.LibWaypointFollower.calcAbsoluteCoordinate(rotate_p, current_pose);
    
    traj_circle_array(idx) = tf_p;
    idx = idx + 1;
end

% reverse vector
traj_circle_array(1:idx-1) = flip(traj_circle_array(1:idx-1));

for rad = 0:-increment:-range
    % calc a point of circumference
    p = blank_msg;
    p.X = radius * cos(rad);
    p.Y = radius * sin(rad);
    
    % transform to (radius,0)
    relative_p = blank_msg;
    relative_p.X = p.X - radius;
    relative_p.Y = p.Y;

    % rotate -90°
    rotate_p = autoware.LibWaypointFollower.rotatePoint(relative_p, -90);
    
    % transform to vehicle plane
    tf_p = autoware.LibWaypointFollower.calcAbsoluteCoordinate(rotate_p, current_pose);
    
    traj_circle_array(idx) = tf_p;
    idx = idx + 1;    
end

% [EOF]

== matlab function pure_pursuit_sl/main_loop/loop_action/canGetCurvature/getNextWaypoint/If Action Subsystem1/MATLAB Function ==
  data: path_size input; next_waypoint_number output int32; current_pose_Pose input; lookahead_distance input; waypoint input
function next_waypoint_number = valid_curve(path_size, current_pose_Pose, lookahead_distance, waypoint)
get_idx = int32(1);

for i = 1:path_size    
    if i == path_size
        disp('search waypoint is the last')
        get_idx = int32(i);
        break;
    end    
    current_pose_2d = [current_pose_Pose.Position.X current_pose_Pose.Position.Y];
    waypoint_2d = [waypoint(i).Pose.Pose.Position.X waypoint(i).Pose.Pose.Position.Y];   
    if norm(current_pose_2d - waypoint_2d) > lookahead_distance
        get_idx = int32(i);
        break;
    end
end
next_waypoint_number = get_idx;

== matlab function pure_pursuit_sl/main_loop/loop_action/canGetCurvature/curvature/check whether curvature is valid or not ==
  data: is_valid_curve output boolean; current_pose_Pose input; minimum_lookahead_distance input; waypoint input
function is_valid_curve = fcn(current_pose_Pose, minimum_lookahead_distance, waypoint)

flag = false;
for i = 1 : length(waypoint)
    current_pose_2d = [current_pose_Pose.Position.X current_pose_Pose.Position.Y];
    waypoint_2d = [waypoint(i).Pose.Pose.Position.X waypoint(i).Pose.Pose.Position.Y];
    if norm(current_pose_2d - waypoint_2d) > minimum_lookahead_distance
        flag = true;
        break;
    end
end
is_valid_curve = flag;

== matlab function pure_pursuit_sl/main_loop/loop_action/VisualizationWithRviz/displayTrajectoryCircle/MATLAB Function ==
  data: colors output Bus: SL_Bus_pure_pursuit_sl_std_msgs_ColorRGBA size=80; blank_msg_color_rgba input
function colors = setColor(blank_msg_color_rgba)
% 

data_size = 80;
colors = repmat(blank_msg_color_rgba, data_size, 1);

white = blank_msg_color_rgba;
white.A = single(1.0);
white.B = single(1.0);
white.R = single(1.0);
white.G = single(1.0);
for idx = 1:data_size
    colors(idx) = white;
end

% [EOF]

== matlab function pure_pursuit_sl/main_loop/warn_messge/MATLAB Function ==
function fcn

disp('Necessary topics are not subscribed yet ... ');

== matlab function pure_pursuit_sl/main_loop/loop_action/canGetCurvature/lost_next_waypoint/MATLAB Function ==
function fcn

disp('lost next waypoint');

== matlab function pure_pursuit_sl/main_loop/loop_action/canGetCurvature/curvature/if is_linear_interpolation_ is false or next waypoint is first or last/If Action Subsystem/MATLAB Function ==
function fcn

disp('lost target! ');

== matlab function pure_pursuit_sl/main_loop/loop_action/canGetCurvature/curvature/if is_linear_interpolation_ is false or next waypoint is first or last/calcCurvature/calcCurvature/calcRelativeCoordinate/inverse_matrix/inverse ==
  data: u input; y output
function y = fcn(u)

y = inv(u);
